simulink model "q1"  (R2026a)
settings: Solver=VariableStepAuto
model workspace (MAT data in the model file):
  K = Simulink.Parameter
  K.Value = 1
  K.Complexity = 'real'
  K.Dimensions = [1 1]
  K.DataType = 'auto'
  a = Simulink.Parameter
  a.Value = 2
  a.Complexity = 'real'
  a.Dimensions = [1 1]
  a.DataType = 'auto'
  k = 5
settings Model: Creator=LAB_PC  LastModifiedBy=LAB_PC

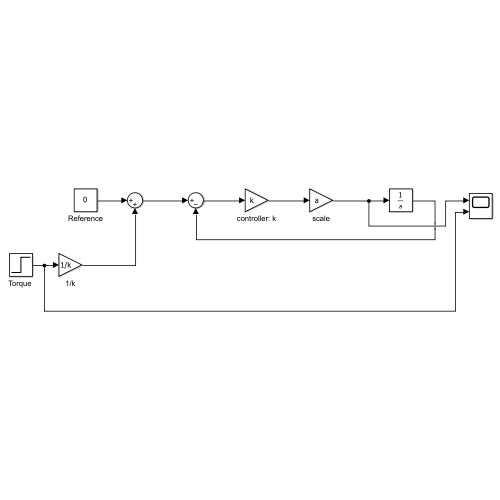
[thumbnail: Simulink's stored preview of the top-level diagram]
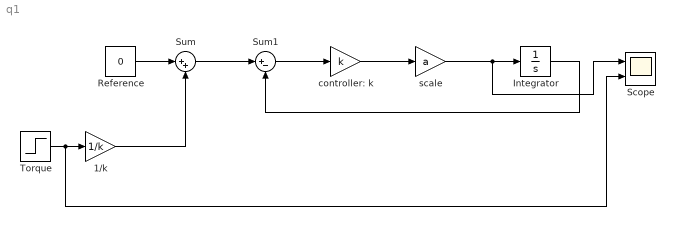
== system q1 ==
  1/k : Gain  Gain=1/k
  Integrator : Integrator
  Reference : Constant  Value=0
  Scope : Scope  NumInputPorts=2
      settings: TimeAxisLabels=None  ActiveDisplayYMinimum=-0.50000000000000044  ActiveDisplayYMaximum=2
  Sum : Sum  Inputs=|++
  Sum1 : Sum  Inputs=|+-
  "Torque " : Step  SampleTime=0
  controller: k : Gain  Gain=k
  scale : Gain  Gain=a
  wires:
  controller: k/1 -> scale/1
  scale/1 -> Scope/1, Integrator/1
  Sum1/1 -> controller: k/1
  Reference/1 -> Sum/1
  1/k/1 -> Sum/2
  "Torque "/1 -> Scope/2, 1/k/1
  Sum/1 -> Sum1/1
  Integrator/1 -> Sum1/2
